simulink model "sauna_sim"  (R2023a)
settings: Solver=VariableStepAuto  StartTime=0.0  StopTime=3600*2  RelTol=1e-3  AbsTol=1e-3
undefined symbols (not defined in the file or in its folder): cost_electricity, cost_gas, gebouw2_temp, gebouw_temp, mean_mean, opgiet_deur_d, opgiet_deur_opp, opgiet_muur_1_hout_d, opgiet_muur_1_isol_d, opgiet_muur_1_opp, opgiet_muur_2_opp, opgiet_muur_3_opp, opgiet_muur_4_opp, opgiet_plafond_opp, opgiet_volume, R_hout, R_hout_plafond, R_isol, R_muur_2_gips, R_muur_3_gips, R_muur_3_raam, R_muur_4_buiten, R_muur_4_gips, R_muur_4_raam, R_opgiet_hout, R_opgiet_isol, R_sauna2_deur, R_se, R_si, rho_lucht, sauna1_deur_d, sauna1_deur_opp, sauna1_muur_1_hout_d, sauna1_muur_1_isol_d, sauna1_muur_1_opp, sauna1_muur_2_gips_d, sauna1_muur_2_opp, sauna1_muur_3_gips_d, sauna1_muur_3_opp, sauna1_muur_4_gips_d, sauna1_muur_4_opp, sauna1_plafond_hout_d, sauna1_plafond_isol_d, sauna1_plafond_opp, sauna1_R_muur_2_gips, sauna1_R_muur_3_gips, sauna1_R_muur_4_gips, sauna1_vol, sauna2_deur_opp, sauna2_muur_1_hout_d, sauna2_muur_1_isol_d, sauna2_muur_1_opp, sauna2_muur_2_gips_d, sauna2_muur_2_opp, sauna2_muur_3_gips_d, sauna2_muur_3_opp, sauna2_muur_3_raam_d, sauna2_muur_3_raam_opp, sauna2_muur_4_gips_d, sauna2_muur_4_opp ... (+6)
libraries: fl_lib x491, nesl_utility x30
(part 6 of 6)

== matlab function sauna_sim/Thermostat ==
  settings: updateMethod=DISCRETE  sampleTime=50
  data: power input; Troom input; heat output; set_temp input
function heat = thermostat(power, Troom, set_temp)
%Implement the thermostat logic for the heating system
%#codegen
    persistent HEAT

    if isempty(HEAT)
        HEAT = false;
    end
    
    if HEAT && (Troom > set_temp || ~power)
        HEAT = false;
    elseif ~HEAT && Troom < set_temp && power
        HEAT = true;
    end
    
    heat = HEAT;
    
end

== matlab function sauna_sim/Thermostat1 ==
  settings: updateMethod=DISCRETE  sampleTime=50
  data: power input; Troom input; heat output; set_temp input
function heat = thermostat(power, Troom, set_temp)
%Implement the thermostat logic for the heating system
%#codegen
    persistent HEAT

    if isempty(HEAT)
        HEAT = false;
    end
    
    if HEAT && (Troom > set_temp || ~power)
        HEAT = false;
    elseif ~HEAT && Troom < set_temp && power
        HEAT = true;
    end
    
    heat = HEAT;
    
end

== matlab function sauna_sim/Thermostat2 ==
  settings: updateMethod=DISCRETE  sampleTime=50
  data: power input; Troom input; heat output; set_temp input
function heat = thermostat(power, Troom, set_temp)
%Implement the thermostat logic for the heating system
%#codegen
    persistent HEAT

    if isempty(HEAT)
        HEAT = false;
    end
    
    if HEAT && (Troom > set_temp || ~power)
        HEAT = false;
    elseif ~HEAT && Troom < set_temp && power
        HEAT = true;
    end
    
    heat = HEAT;
    
end

== matlab function sauna_sim/Thermostat Gebouw ==
  settings: updateMethod=DISCRETE  sampleTime=50
  data: power input; Troom input; heat output; set_temp input
function heat = thermostat(power, Troom, set_temp)
%Implement the thermostat logic for the heating system
%#codegen
    persistent HEAT

    if isempty(HEAT)
        HEAT = false;
    end
    
    if HEAT && (Troom > set_temp || ~power)
        HEAT = false;
    elseif ~HEAT && Troom < set_temp && power
        HEAT = true;
    end
    
    heat = HEAT;
    
end
